simulink model "simscheme"  (R2021a)
settings: Solver=FixedStepAuto  StartTime=0.0  StopTime=250  FixedStep=T_s  RelTol=1e-3
values from neighbouring files (symbols this model uses):
  K1 = W1 / X    [LPVGainScheduling.m]
  K2 = W2 / X    [LPVGainScheduling.m]
  K3 = W3 / X    [LPVGainScheduling.m]
  K4 = W4 / X    [LPVGainScheduling.m]
  T_s = 0.1    [main.m]
  x0 = [-30;0;0]    [main.m]
settings Model: PacingRate=1000  Creator=nicol  LastModifiedBy=nicol

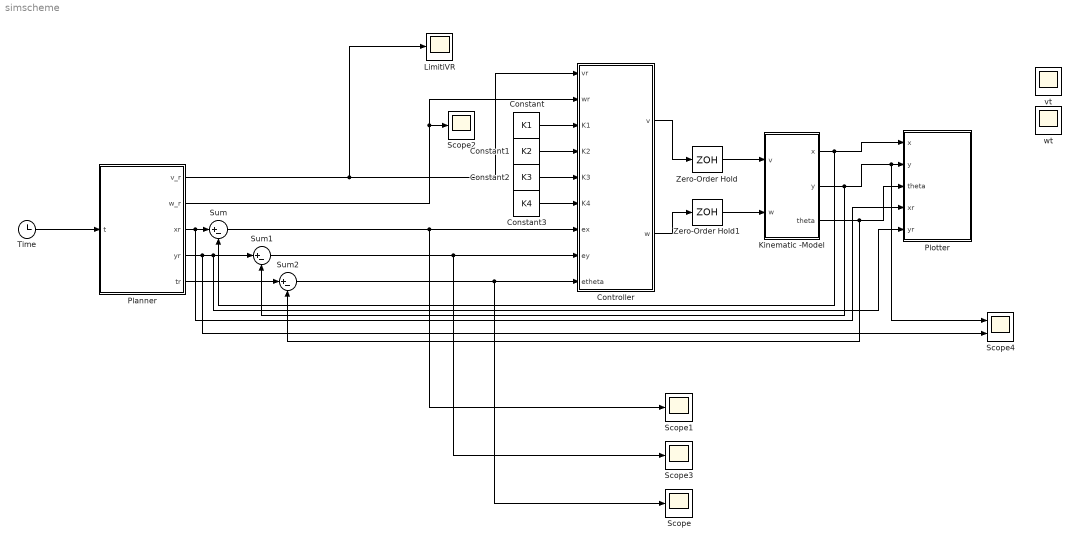
== system simscheme ==
  Constant : Constant  Value=K1
  Constant1 : Constant  Value=K2
  Constant2 : Constant  Value=K3
  Constant3 : Constant  Value=K4
  Controller : MATLAB Function  TreatAsAtomicUnit=on
  Kinematic -Model : Subsystem
  LimitiVR : Scope
  Planner : MATLAB Function  TreatAsAtomicUnit=on
  Plotter : MATLAB Function  TreatAsAtomicUnit=on
  Scope{,1..3} (4 alike) : Scope
  Scope4 : Scope  NumInputPorts=2
  Sum : Sum  Inputs=|+-
  Sum1 : Sum  Inputs=|+-
  Sum2 : Sum  Inputs=|+-
  Time : Clock
  Zero-Order Hold : ZeroOrderHold  SampleTime=T_s
  Zero-Order Hold1 : ZeroOrderHold  SampleTime=T_s
  vt : Scope
  wt : Scope
  wires:
  Time/1 -> Planner/1(t)
  Planner/3(xr) -> Plotter/4(xr), Sum/1
  Planner/4(yr) -> Scope4/2, Plotter/5(yr), Sum1/1
  Planner/5(tr) -> Sum2/1
  Sum2/1 -> Scope/1, Controller/9(etheta)
  Sum/1 -> Scope1/1, Controller/7(ex)
  Planner/2(w_r) -> Controller/2(wr), Scope2/1
  Constant/1 -> Controller/3(K1)
  Constant1/1 -> Controller/4(K2)
  Constant2/1 -> Controller/5(K3)
  Constant3/1 -> Controller/6(K4)
  Sum1/1 -> Scope3/1, Controller/8(ey)
  Planner/1(v_r) -> LimitiVR/1, Controller/1(vr)
  Zero-Order Hold/1 -> Kinematic -Model/1(v)
  Zero-Order Hold1/1 -> Kinematic -Model/2(w)
  Controller/1(v) -> Zero-Order Hold/1
  Controller/2(w) -> Zero-Order Hold1/1
  Kinematic -Model/1(x) -> Sum/2, Plotter/1(x)
  Kinematic -Model/2(y) -> Scope4/1, Plotter/2(y), Sum1/2
  Kinematic -Model/3(theta) -> Sum2/2, Plotter/3(theta)

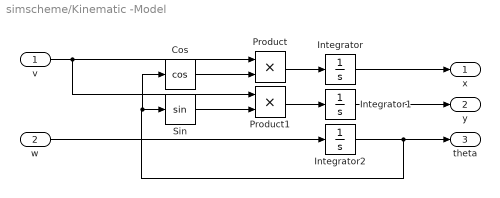
== system simscheme/Kinematic -Model ==
  v : Inport
  w : Inport  Port=2
  Cos : Trigonometry  Operator=cos
  Integrator : Integrator  InitialCondition=x0(1)
  Integrator1 : Integrator  InitialCondition=x0(2)
  Integrator2 : Integrator  InitialCondition=x0(3)
  Product : Product
  Product1 : Product
  Sin : Trigonometry
  x : Outport
  y : Outport  Port=2
  theta : Outport  Port=3
  wires:
  v/1 -> Product1/1, Product/1
  Integrator2/1 -> theta/1, Cos/1, Sin/1
  Sin/1 -> Product1/2
  Integrator/1 -> x/1
  w/1 -> Integrator2/1
  Product1/1 -> Integrator1/1
  Integrator1/1 -> y/1
  Product/1 -> Integrator/1
  Cos/1 -> Product/2

== matlab function simscheme/Planner ==
  data: t input; v_r output; w_r output; xr output; yr output; tr output
function [v_r,w_r,xr,yr,tr] = getTraj(t)
A =5;
w =0.1;
% if(t >= 60 && t <= 150)
%     A = 10;
% elseif(t>150 && t <= 210)
%     A = 15;
% elseif(t > 210)
%     A = 20;
% end
% definizione ingressi sfruttando la piattezza differenziale
xr    =   t;
yr    =   A*sin(w*t)+A*sin(2*w*t);
% derivata prima
x_d   =   1;
y_d   =   A*cos(w*t)*w+2*A*cos(2*w*t)*w;
tr    = atan2(y_d,x_d);
% derivata seconda
x_dd =  0;
y_dd =  -A*sin(w*t)*w*w-4*A*sin(2*w*t)*w*w;
% definizione ingressi corrispondenti
v_r  = sqrt(x_d*x_d + y_d*y_d);
w_r  = (y_dd*x_d - x_dd*y_d)/(x_d*x_d + y_d*y_d);
end

== matlab function simscheme/Plotter ==
  settings: updateMethod=DISCRETE
  data: x input; y input; theta input; xr input; yr input
function plotDD(x,y,theta,xr,yr)
persistent xp yp xrr yrr
if(isempty(xp))
    xp  = [];
    yp  = [];
    xrr = [];
    yrr = [];
end
% Definizione Parametri Strutturali Robot
W = 2;                    % Base triangolo
H = 1.7;                  % Altezza triangolo
coder.extrinsic("patch");
% Definizione Robot -> Struttura Geometrica : Triangolo
vertici_triangolo  = [-W/2 W/2 -W/2; 
                      -H/2  0  +H/2;
                        0   0    0];
% Defizione Matrice in SO(3) -> Rotazione Rispetto all'asse z
R = [cos(theta) ,   -sin(theta) , 0;
     sin(theta) ,  cos(theta) , 0;
         0      ,       0     , 1];
% Rotazione Dei Vettori Posizione Vertici Differential Drive
rotazione   = R*vertici_triangolo;
% Traslazione
traslazione = [x , x , x;
               y , y , y;
               0 , 0 , 0];
% memorizzazione
xp  = [xp , x];
yp  = [yp , y];
xrr = [xrr , xr];
yrr = [yrr , yr];
% Posa := Traslazione + Rotazione
posa        = traslazione + rotazione;
% Apertura Finestra Di Disegno
clf;
hold on;
grid on;
axis square;
xlim([-50, 270]);
ylim([-15, 15]);
% Rappresentazione Robot
patch([posa(1,:)],[posa(2,:)],[posa(3,:)],'r');
plot(xp,yp,'b--');
plot(xrr,yrr,'r--');
end

== matlab function simscheme/Controller ==
  data: v output; w output; vr input; wr input; K1 input; K2 input; K3 input; K4 input; ex input; ey input; etheta input
function [v,w] = control(vr,wr,K1,K2,K3,K4,ex,ey,etheta)
% definizione limiti 
vMin =    1;
vMax =    5;
wMin =   -5;
wMax =    5;
% Controllo Gain Scheduling
p1   = ((vr-vMin)/(vMax-vMin))*((wr -wMin)/(wMax - wMin));
p2   = ((vr - vMin)/(vMax-vMin))*((wMax-wr)/(wMax - wMin));
p3   = ((vMax-vr)/(vMax-vMin))*((wMax-wr)/(wMax -wMin));
p4   = ((vMax-vr)/(vMax-vMin))*((wr -wMin)/(wMax -wMin));
% Guadagno Controllore Gain Scheduling
K    = p1*K1+p2*K2+p3*K3+p4*K4;
% Definizione ingressi Addizionali
u1   = K(1,1)*ex+K(1,2)*ey+K(1,3)*etheta;
u2   = K(2,1)*ex+K(2,2)*ey+K(2,3)*etheta;
% Ingressi Effettivi
v    = vr*cos(etheta)-u1;
w    = wr - u2;
end
